simulink model "becslo"  (R2013b)
settings: Solver=FixedStepDiscrete  SolverMode=SingleTasking  StartTime=0.0  StopTime=inf  FixedStep=0.01  RelTol=1e-3
undefined symbols (not defined in the file or in its folder): A, N
libraries: xbsIndex_r4 x6, simulink x2, JTAGRuntimeCosim_r4 x1
settings Model: Creator=laca  LastModifiedBy=laca

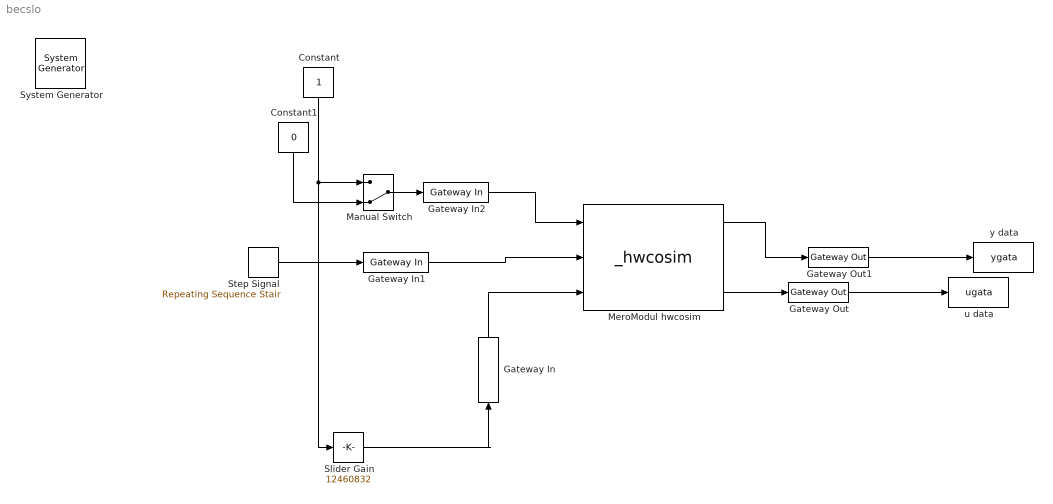
== system becslo ==
  " System Generator" : xbsIndex_r4/ System Generator  Tag=genX  xilinxfamily=spartan3e  part=xc3s500e  speed=-4  package=pq208  synthesis_tool=XST  clock_wrapper=Clock Enables  directory=./netlist  proj_type=Project Navigator  Synth_file=XST Defaults  Impl_file=ISE Defaults  testbench=off  simulink_period=1  sysclk_period=20  dcm_input_clock_period=10  incr_netlist=off  trim_vbits=Everywhere in SubSystem  dbl_ovrd=According to Block Masks  core_generation=According to Block Masks  run_coregen=off  deprecated_control=off  eval_field=0  block_type=sysgen
  Constant : Constant
  Constant1 : Constant  Value=0
  Gateway In : xbsIndex_r4/Gateway In  gui_display_data_type=Fixed-point  arith_type=Unsigned  n_bits=24  bin_pt=0  preci_type=Single  exp_width=8  frac_width=24  quantization="Round  (unbiased: +/- Inf)"  overflow=Saturate  period=1  dbl_ovrd=off  timing_constraint=None  locs_specified=off  LOCs={}  UseAsADC=off  ADCChannel='1'  inherit_from_input=off  hdl_port=on  block_type=gatewayin
  Gateway In1 : xbsIndex_r4/Gateway In  gui_display_data_type=Fixed-point  arith_type="Signed  (2's comp)"  n_bits=17  bin_pt=0  preci_type=Single  exp_width=8  frac_width=24  quantization="Round  (unbiased: +/- Inf)"  overflow=Saturate  period=1  dbl_ovrd=off  timing_constraint=None  locs_specified=off  LOCs={}  UseAsADC=off  ADCChannel='1'  inherit_from_input=off  hdl_port=on  block_type=gatewayin
  Gateway In2 : xbsIndex_r4/Gateway In  gui_display_data_type=Boolean  arith_type=Boolean  n_bits=16  bin_pt=14  preci_type=Single  exp_width=8  frac_width=24  quantization="Round  (unbiased: +/- Inf)"  overflow=Saturate  period=1  dbl_ovrd=off  timing_constraint=None  locs_specified=off  LOCs={}  UseAsADC=off  ADCChannel='1'  inherit_from_input=off  hdl_port=on  block_type=gatewayin
  Gateway Out : xbsIndex_r4/Gateway Out  inherit_from_input=off  hdl_port=on  timing_constraint=None  locs_specified=off  LOCs={}  UseAsDAC=off  DACChannel='1'  block_type=gatewayout
  Gateway Out1 : xbsIndex_r4/Gateway Out  inherit_from_input=off  hdl_port=on  timing_constraint=None  locs_specified=off  LOCs={}  UseAsDAC=off  DACChannel='1'  block_type=gatewayout
  Manual Switch : ManualSwitch  CurrentSetting=0
  MeroModul hwcosim : JTAGRuntimeCosim_r4/_hwcosim  clkSrc=Free Running  hasCombinationalPath=off  bitfileName=C:\Users\laca\Desktop\iRoobo2014Ver3\Fpga\SPARTAN3E\Spartan3E6500SystemVer2\MeresEsRendszerBecsles\netlist\meromodul_cw.bit  skipConfig=off  cable=Auto Detect  speed=N/A  cablePort=N/A  cableLocation=Local  shareCable=off  enable_codebug=on  design_xtable=|  engineDll=JTAGCosimEngine.dll  cableWaitTime=10  bscanPos=1  IRLengths=[6,8]  useWaitBox=1  hasBufgmux=on  Scheme=Cosim  useCmdProc=1  hasProc=0  useImpact=0  printLogFile=0  block_type=jtagcosim
      | {
      |   'clkWrapper' => 'meromodul_cw',
      |   'clocksGcd' => undef,
      |   'device' => 'xc3s500e-4pq208',
      |   'ports' => {
      |     'enapwm' => {
      |       'bd_port_index' => 0,
      |       'direction' => 'in',
      |       'icon_text' => 'enaPWM',
      |       'period' => 1,
      |       'sim_pause_trigger' => false,
      |       'type' => 'Bool',
      |       'width' => 1,
      |     },
      |     'position' => {
      |       'bd_port_index' => 0,
      |       'direction' => 'out',
      |       'icon_text' => 'position',
      |       'period' => 1,
      |       'sim_pause_trigger' => false,
      |       'type' => 'Fix_16_0',
      |       'width' => 16,
      |     },
      |     'speed' => {
      |       'bd_port_index' => 1,
      |       'direction' => 'out',
      |       'icon_text' => 'speed',
      |       'period' => 1,
      |       'sim_pause_trigger' => false,
      |       'type' => 'Fix_16_0',
      |       'width' => 16,
      |     },
      |     'step' => {
      |       'bd_port_index' => 1,
      |       'direction' => 'in',
      |       'icon_text' => 'Step',
      |       'period' => 1,
      |       'sim_pause_trigger' => false,
      |       'type' => 'Fix_17_0',
      |       'width' => 17,
      |     },
      |     'tsvalue' => {
      |       'bd_port_index' => 2,
      |       'direction' => 'in',
      |       'icon_text' => 'TsValue',
      |       'period' => 1,
      |       'sim_pause_trigger' => false,
      |       'type' => 'UFix_24_0',
      |       'width' => 24,
      |     },
      |     'uout' => {
      |       'bd_port_index' => 2,
      |       'direction' => 'out',
      |       'icon_text' => 'Uout',
      |       'period' => 1,
      |       'sim_pause_trigger' => false,
      |       'type' => 'UFix_16_0',
      |       'width' => 16,
      |     },
      |   },
      |   'shared_memories' => {},
      | }
  Slider Gain : simulink/Math Operations/Slider Gain  low=0  gain=12460832  high=16000000
  Step Signal : simulink/Sources/Repeating Sequence Stair  OutValues=[100 1000 10000 20000 ].'  tsamp=1000  OutMin=[]  OutMax=[]  OutDataTypeStr=double  OutputDataTypeScalingMode=double  OutDataType=fixdt(0,8)  ConRadixGroup=Best Precision: Vector-wise  OutScaling=2^-12
  u data : ToWorkspace  VariableName=ugata  SampleTime=1
  y data : ToWorkspace  VariableName=ygata  SampleTime=1
  wires:
  Step Signal/1 -> Gateway In1/1
  MeroModul hwcosim/3 -> Gateway Out/1
  Constant/1 -> Slider Gain/1, Manual Switch/1
  Slider Gain/1 -> Gateway In/1
  Manual Switch/1 -> Gateway In2/1
  Constant1/1 -> Manual Switch/2
  Gateway In/1 -> MeroModul hwcosim/3
  Gateway In1/1 -> MeroModul hwcosim/2
  Gateway In2/1 -> MeroModul hwcosim/1
  Gateway Out/1 -> u data/1
  Gateway Out1/1 -> y data/1
  MeroModul hwcosim/1 -> Gateway Out1/1
